simulink model "untitled"  (R2021b)
settings: Solver=VariableStepAuto  StartTime=0.0  StopTime=10.0  RelTol=1e-3
settings Model: Creator=stav  LastModifiedBy=stav

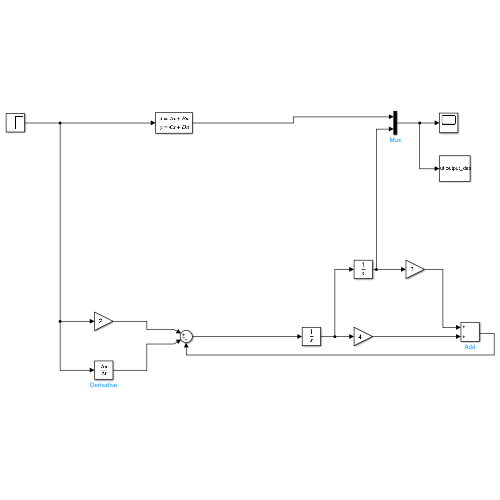
[thumbnail: Simulink's stored preview of the top-level diagram]
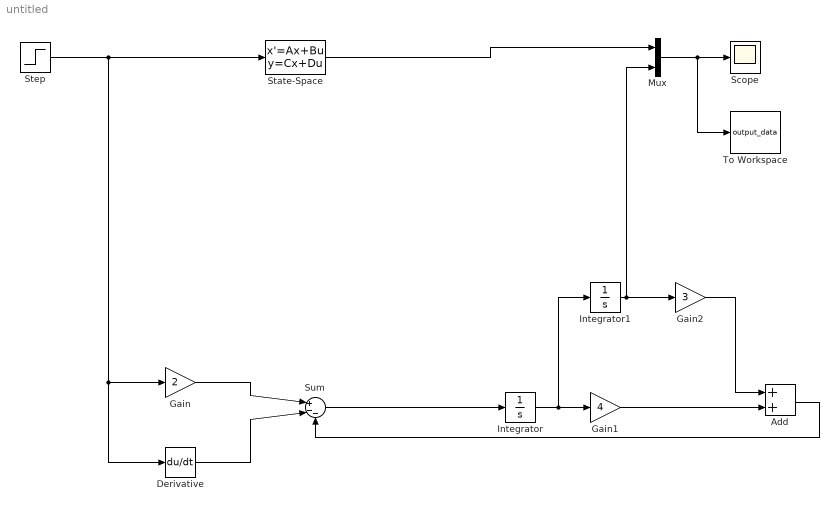
== system untitled ==
  Add : Sum
  Derivative : Derivative
  Gain : Gain  Gain=2
  Gain1 : Gain  Gain=4
  Gain2 : Gain  Gain=3
  Integrator : Integrator  InitialCondition=1
  Integrator1 : Integrator
  Mux : Mux  Inputs=2
  Scope : Scope
  State-Space : StateSpace  A=[-4 1; -3 0]  B=[-1; 2]  C=[1 0]  D=0  InitialCondition=[0.5; 0]
  Step : Step  Time=0  SampleTime=0
  Sum : Sum  Inputs=|+--
  To Workspace : ToWorkspace  VariableName=output_data  SampleTime=-1
  wires:
  Step/1 -> State-Space/1, Derivative/1, Gain/1
  Gain/1 -> Sum/1
  Derivative/1 -> Sum/2
  Sum/1 -> Integrator/1
  Integrator/1 -> Integrator1/1, Gain1/1
  Add/1 -> Sum/3
  Gain1/1 -> Add/2
  Integrator1/1 -> Mux/2, Gain2/1
  Gain2/1 -> Add/1
  State-Space/1 -> Mux/1
  Mux/1 -> To Workspace/1, Scope/1
